simulink model "PubIfDecisionTOS_MDL"  (R2020b)
settings: configuration reference "DspaceConfig" (kept outside this file)
PostLoadFcn:
  | if any(exist('dsrtsu_mdlpostloadfcn', 'file') ~= 0), dsrtsu_mdlpostloadfcn('Execute', bdroot); end
InitFcn:
  | , if any(exist('dsmpb_private', 'file') ~= 0), dsmpb_private('dsmpb_mdlclblib', 'Init', bdroot); end,
undefined symbols (not defined in the file or in its folder): C_TOS_ACCEgoRAxletoFbumplength_m, C_TOS_ACCTargetFront_Flag, C_TOS_AEBJAPedObjDxThre_Val, C_TOS_AEBJAPedObjDyThre_Val, C_TOS_AEBJATargetSize_Val, C_TOS_AEBJAVehObjDxThre_Val, C_TOS_AEBJAVehObjDyThre_Val, C_TOS_AEBJuncPedTargetSize_Val, C_TOS_AEBLatObjDxThre_Val, C_TOS_AEBLatPedDyThre_Val, C_TOS_AEBLatTargetSize_Val, C_TOS_AEBLongTargetInEgoFront_Flag, C_TOS_axAbsGround_Parameter, C_TOS_CameraConfirmedFlag, C_TOS_CNsubjWidth, C_TOS_CurrentLaneCoreMinWidth_Val, C_TOS_CutInProb_Val_Zero, C_TOS_CutOutProb_Val_Zero, C_TOS_D2R_Val, C_TOS_DefaultValueObjectToCenterLine_dy, C_TOS_EgoCarWidth_Val, C_TOS_EgoDxRefPoint_m, C_TOS_EgoRAxletoFbumplength_m, C_TOS_HalfWidthVehicle_Con, C_TOS_HWA_CurrentLaneFlag, C_TOS_HWA_LeftLaneFlag, C_TOS_HWA_MovingDir_Vaild, C_TOS_HWA_MovState_Vaild, C_TOS_HWA_RightLaneFlag, C_TOS_LaneLineCourseErrorFront, C_TOS_LaneLineCourseErrorRear, C_TOS_MotorbikeDefaultWidth_m, C_TOS_NumberOfEffectiveTargets, C_TOS_Obj_Age_Val, C_TOS_Objdx_Constraint_Val, C_TOS_ObjectDefaultWidth_m, C_TOS_ObjInCurrentLane_Val, C_TOS_ObjInCurrentLaneValid, C_TOS_ObjInLeftLaneValid, C_TOS_ObjInRightLaneValid, C_TOS_ObjNotInCurrentLane_Val, C_TOS_ObjNotREElementType, C_TOS_ObjPredictDis_dy_ConstantVal_Zeros, C_TOS_ObjToCenterLine_ConstantVal_Zeros, C_TOS_OFMObjIDInvilad_Val, C_TOS_PIL_LatDisCons_Val_zero, C_TOS_PIL_ObjectCutInFlag_b, C_TOS_PIL_ObjectCutOutFlag_b, C_TOS_PIL_ObjLaneProb_al_Val, C_TOS_PP_ObjFusType_FC_Confirm_b, C_TOS_PP_ObjFusType_FC_FR_Confirm_b, C_TOS_PP_ObjFusType_FR_Confirm_b, C_TOS_RE_80BoolDefault_Val, C_TOS_RE_80Single181Default_Val, C_TOS_RE_80Single255Default_Val, C_TOS_RE_80Uint8Default_Val, C_TOS_RE_D2R, C_TOS_RE_D_180_Val, C_TOS_RE_InvalidObjectID_Val, C_TOS_RE_InvalidTargetChainDir_Val ... (+142)
libraries: simulink x1650, TOS_LIB x361, canfdmsglib x14
(part 3 of 69)

== system PubIfDecisionTOS_MDL/TOS_20201112/TOS_2012080320/Subsystem2 ==
  TOS_ACCP0 : Inport
  TOS_ACCP1 : Inport  Port=2
  TOS_ACCP2 : Inport  Port=3
  TOS_ACCP3 : Inport  Port=4
  TOS_ACC4 : Inport  Port=5
  TOS_ACCP5 : Inport  Port=6
  Bus Selector : BusSelector  OutputSignals=ACCTgtObjAy,ACCTgtObjCntAlive,ACCTgtObjExist,ACCTgtObjObstcl,ACCTgtObjVy,IDP0,ObjDYP0,ObjMovingStateP0,ObjTypeP0,Object_Orientation,P0CutInflg,P0HeadingAngle,axAbsGroundP0,dxP0,fu_typeP0,rangeP0,targetExistP0,vxRelP0
  Bus Selector1 : BusSelector  OutputSignals=IDP1,ObjDYP1,ObjMovingStateP1,ObjTypeP1,P1HeadingAngle,axAbsGroundP1,dxP1,fu_typeP1,rangeP1,targetExistP1,vxRelP1
  Bus Selector2 : BusSelector  OutputSignals=IDP2,ObjDYP2,ObjMovingStateP2,ObjTypeP2,P2CutinProb,P2HeadingAngle,axAbsGroundP2,dxP2,fu_typeP2,rangeP2,targetExistP2,vxRelP2
  Bus Selector3 : BusSelector  OutputSignals=IDP3,ObjDYP3,ObjMovingStateP3,ObjTypeP3,P3CutinProb,P3HeadingAngle,axAbsGroundP3,dxP3,fu_typeP3,rangeP3,targetExistP3,vxRelP3
  Bus Selector4 : BusSelector  OutputSignals=ObjTypeP4,dxP4,dyP4,targetExistP4
  Bus Selector5 : BusSelector  OutputSignals=ObjTypeP5,dxP5,dyP5,targetExistP5
  CAN FD Pack : canfdmsglib/CAN FD Pack  CANdbFile=F:\InternalData03_ACC_AEBLog_ELK_LC_LCKie_20200927.dbc  MsgList=(none)  MsgName=TOS_ACC_P0  ProtocolMode=CAN FD  MsgIDType=Standard (11-bit identifier)  MsgIdentifier=512  MsgLength=64  Remote=off  BRSSwitch=off  ApplyMinMax=off  SignalInfo={'{'P0_ACCTgtObjAy','12','12','BE','signed','Standard','0','0.01','0','-20.48','20.47';'P0_ACCTgtObjCntAlive','16','8','BE','unsigned','Standard','0','1','0','0','255';'P0_ACCTgtObjExist','24','8','BE','unsigned','Standard','0','0.01','0','0','2.55';'P0_ACCTgtObjObstcl','46','10','BE','unsigned','Standard','0','0.001','0','0','1.023';'P0_ACCTgtObjVy','58','14','BE','signed','Standard','0','0.01','0','-81.92','81.91';'P0_IDP0','96','8','BE','unsigned','Standard','0','1','0','0','255';'P0_ObjDYP0','114','14','BE','signed','Standard','0','0.005','0','-40.96','40.955';'P0_ObjMovingStateP0','122','6','BE','unsigned','Standard','0','1','0','0','63';'P0_ObjTypeP0','72','4','BE','unsigned','Standard','0','1','0','0','15';'P0_Object_Orientation','8','4','BE','unsigned','Standard','0','1','0','0','15';'P0_P0CutInflg','57','1','BE','unsigned','Standard','0','1','0','0','1';'P0_P0HeadingAngle','128','8','BE','unsigned','Standard','0','0.0041','0','0','1.0455';'P0_axAbsGroundP0','76','12','BE','signed','Standard','0','0.01','0','-20.48','20.47';'P0_dxP0','89','15','BE','unsigned','Standard','0','0.0063','0','0','206.4321';'P0_fu_typeP0','40','6','BE','unsigned','Standard','0','1','0','0','63';'P0_rangeP0','145','15','BE','unsigned','Standard','0','0.01','0','0','327.67';'P0_targetExistP0','56','1','BE','unsigned','Standard','0','1','0','0','1'}
      settings: SourceProductBaseCode=VN  DataFormat=CANdb specified signals
  CAN FD Pack1 : canfdmsglib/CAN FD Pack  CANdbFile=F:\InternalData03_ACC_AEBLog_ELK_LC_LCKie_20200927.dbc  MsgList=(none)  MsgName=TOS_ACC_P1_P2_P3_P4_P5  ProtocolMode=CAN FD  MsgIDType=Standard (11-bit identifier)  MsgIdentifier=513  MsgLength=64  Remote=off  BRSSwitch=off  ApplyMinMax=off  SignalInfo={'{'P1_IDP1','16','8','BE','unsigned','Standard','0','1','0','0','255';'P1_ObjDYP1','58','14','BE','signed','Standard','0','0.005','0','-40.96','40.955';'P1_ObjMovingStateP1','66','6','BE','unsigned','Standard','0','1','0','0','63';'P1_ObjTypeP1','32','4','BE','unsigned','Standard','0','1','0','0','15';'P1_P1HeadingAngle','72','8','BE','unsigned','Standard','0','0.0041','0','0','1.0455';'P1_axAbsGroundP1','36','12','BE','signed','Standard','0','0.01','0','-20.48','20.47';'P1_dxP1','9','15','BE','unsigned','Standard','0','0.0063','0','0','206.4321';'P1_fu_typeP1','42','6','BE','unsigned','Standard','0','1','0','0','63';'P1_rangeP1','89','15','BE','unsigned','Standard','0','0.0063','0','0','206.4321';'P1_targetExistP1','8','1','BE','unsigned','Standard','0','1','0','0','1';'P1_vxRelP1','104','16','BE','signed','Standard','0','0.00616','0','-201.8509','201.8447';'P2_IDP2','152','8','BE','unsigned','Standard','0','1','0','0','255';'P2_ObjDYP2','170','14','BE','signed','Standard','0','0.005','0','-40.96','40.955';'P2_ObjMovingStateP2','178','6','BE','unsigned','Standard','0','1','0','0','63';'P2_ObjTypeP2','120','4','BE','unsigned','Standard','0','1','0','0','15';'P2_P2CutinProb','184','8','BE','unsigned','Standard','0','0.005','0','0','1.275';'P2_P2HeadingAngle','192','8','BE','unsigned','Standard','0','0.0041','0','0','1.0455';'P2_axAbsGroundP2','124','12','BE','signed','Standard','0','0.01','0','-20.48','20.47';'P2_dxP2','137','15','BE','unsigned','Standard','0','0.0063','0','0','206.4321';'P2_fu_typeP2','146','6','BE','unsigned','Standard','0','1','0','0','63';'P2_rangeP2','209','15','BE','unsigned','Standard','0','0.0063','0','0','206.4321';'P2_targetExistP2','41','1','BE','unsigned','Standard','0','1','0','0','1';'P2_vxRelP2','232','16','BE','signed','Standard','0','0.00616','0','-201.8509','201.8447';'P3_IDP3','272','8','BE','unsigned','Standard','0','1','0','0','255';'P3_ObjDYP3','290','14','BE','signed','Standard','0','0.005','0','-40.96','40.955';'P3_ObjMovingStateP3','298','6','BE','unsigned','Standard','0','1','0','0','63';'P3_ObjTypeP3','248','4','BE','unsigned','Standard','0','1','0','0','15';'P3_P3CutinProb','304','8','BE','unsigned','Standard','0','0.005','0','0','1.275';'P3_P3HeadingAngle','312','8','BE','unsigned','Standard','0','0.0041','0','0','1.0455';'P3_axAbsGroundP3','252','12','BE','signed','Standard','0','0.01','0','-20.48','20.47';'P3_dxP3','265','15','BE','unsigned','Standard','0','0.0063','0','0','206.4321';'P3_fu_typeP3','218','6','BE','unsigned','Standard','0','1','0','0','63';'P3_rangeP3','329','15','BE','unsigned','Standard','0','0.0063','0','0','206.4321';'P3_targetExistP3','40','1','BE','unsigned','Standard','0','1','0','0','1';'P3_vxRelP3','344','16','BE','signed','Standard','0','0.00616','0','-201.8509','201.8447';'P4_ObjTypeP4','376','4','BE','unsigned','Standard','0','1','0','0','15';'P4_dxP4','361','15','BE','unsigned','Standard','0','0.0063','0','0','206.4321';'P4_dyP4','380','12','BE','signed','Standard','0','0.01','0','-20.48','20.47';'P4_targetExistP4','57','1','BE','unsigned','Standard','0','1','0','0','1';'P5_ObjTypeP5','408','4','BE','unsigned','Standard','0','1','0','0','15';'P5_dxP5','393','15','BE','unsigned','Standard','0','0.0063','0','0','206.4321';'P5_dyP5','412','12','BE','signed','Standard','0','0.01','0','-20.48','20.47'}
      settings: SourceProductBaseCode=VN  DataFormat=CANdb specified signals
  TOS_ACCP0_Msg : Outport
  TOS_ACCP1_P2_P3_P4_P5_Msg : Outport  Port=2
  wires:
  TOS_ACCP2/1 -> Bus Selector2/1
  TOS_ACCP1/1 -> Bus Selector1/1
  TOS_ACCP0/1 -> Bus Selector/1
  CAN FD Pack/1 -> TOS_ACCP0_Msg/1
  TOS_ACCP3/1 -> Bus Selector3/1
  TOS_ACC4/1 -> Bus Selector4/1
  TOS_ACCP5/1 -> Bus Selector5/1
  Bus Selector/1 -> CAN FD Pack/1  "<ACCTgtObjAy>"
  Bus Selector/2 -> CAN FD Pack/2  "<ACCTgtObjCntAlive>"
  Bus Selector/3 -> CAN FD Pack/3  "<ACCTgtObjExist>"
  Bus Selector/4 -> CAN FD Pack/4  "<ACCTgtObjObstcl>"
  Bus Selector/5 -> CAN FD Pack/5  "<ACCTgtObjVy>"
  Bus Selector/6 -> CAN FD Pack/6  "<IDP0>"
  Bus Selector/7 -> CAN FD Pack/7  "<ObjDYP0>"
  Bus Selector/8 -> CAN FD Pack/8  "<ObjMovingStateP0>"
  Bus Selector/9 -> CAN FD Pack/9  "<ObjTypeP0>"
  Bus Selector/10 -> CAN FD Pack/10  "<Object_Orientation>"
  Bus Selector/11 -> CAN FD Pack/11  "<P0CutInflg>"
  Bus Selector/12 -> CAN FD Pack/12  "<P0HeadingAngle>"
  Bus Selector/13 -> CAN FD Pack/13  "<axAbsGroundP0>"
  Bus Selector/14 -> CAN FD Pack/14  "<dxP0>"
  Bus Selector/15 -> CAN FD Pack/15  "<fu_typeP0>"
  Bus Selector/16 -> CAN FD Pack/16  "<rangeP0>"
  Bus Selector/17 -> CAN FD Pack/17  "<targetExistP0>"
  Bus Selector/18 -> CAN FD Pack/18  "<vxRelP0>"
  Bus Selector1/4 -> CAN FD Pack1/4  "<ObjTypeP1>"
  Bus Selector1/5 -> CAN FD Pack1/5  "<P1HeadingAngle>"
  Bus Selector1/3 -> CAN FD Pack1/3  "<ObjMovingStateP1>"
  Bus Selector1/6 -> CAN FD Pack1/6  "<axAbsGroundP1>"
  Bus Selector1/2 -> CAN FD Pack1/2  "<ObjDYP1>"
  Bus Selector1/7 -> CAN FD Pack1/7  "<dxP1>"
  Bus Selector1/1 -> CAN FD Pack1/1  "<IDP1>"
  Bus Selector1/8 -> CAN FD Pack1/8  "<fu_typeP1>"
  Bus Selector1/9 -> CAN FD Pack1/9  "<rangeP1>"
  Bus Selector1/10 -> CAN FD Pack1/10  "<targetExistP1>"
  Bus Selector1/11 -> CAN FD Pack1/11  "<vxRelP1>"
  Bus Selector2/4 -> CAN FD Pack1/15  "<ObjTypeP2>"
  Bus Selector2/5 -> CAN FD Pack1/16  "<P2CutinProb>"
  Bus Selector2/3 -> CAN FD Pack1/14  "<ObjMovingStateP2>"
  Bus Selector2/6 -> CAN FD Pack1/17  "<P2HeadingAngle>"
  Bus Selector2/2 -> CAN FD Pack1/13  "<ObjDYP2>"
  Bus Selector2/7 -> CAN FD Pack1/18  "<axAbsGroundP2>"
  Bus Selector2/1 -> CAN FD Pack1/12  "<IDP2>"
  Bus Selector2/8 -> CAN FD Pack1/19  "<dxP2>"
  Bus Selector2/9 -> CAN FD Pack1/20  "<fu_typeP2>"
  Bus Selector2/10 -> CAN FD Pack1/21  "<rangeP2>"
  Bus Selector2/11 -> CAN FD Pack1/22  "<targetExistP2>"
  Bus Selector2/12 -> CAN FD Pack1/23  "<vxRelP2>"
  Bus Selector3/1 -> CAN FD Pack1/24  "<IDP3>"
  Bus Selector3/2 -> CAN FD Pack1/25  "<ObjDYP3>"
  Bus Selector3/3 -> CAN FD Pack1/26  "<ObjMovingStateP3>"
  Bus Selector3/4 -> CAN FD Pack1/27  "<ObjTypeP3>"
  Bus Selector3/5 -> CAN FD Pack1/28  "<P3CutinProb>"
  Bus Selector3/6 -> CAN FD Pack1/29  "<P3HeadingAngle>"
  Bus Selector3/7 -> CAN FD Pack1/30  "<axAbsGroundP3>"
  Bus Selector3/8 -> CAN FD Pack1/31  "<dxP3>"
  Bus Selector3/9 -> CAN FD Pack1/32  "<fu_typeP3>"
  Bus Selector3/10 -> CAN FD Pack1/33  "<rangeP3>"
  Bus Selector3/11 -> CAN FD Pack1/34  "<targetExistP3>"
  Bus Selector3/12 -> CAN FD Pack1/35  "<vxRelP3>"
  Bus Selector4/3 -> CAN FD Pack1/38  "<dyP4>"
  Bus Selector4/2 -> CAN FD Pack1/37  "<dxP4>"
  Bus Selector4/4 -> CAN FD Pack1/39  "<targetExistP4>"
  Bus Selector4/1 -> CAN FD Pack1/36  "<ObjTypeP4>"
  Bus Selector5/1 -> CAN FD Pack1/40  "<ObjTypeP5>"
  Bus Selector5/2 -> CAN FD Pack1/41  "<dxP5>"
  Bus Selector5/3 -> CAN FD Pack1/42  "<dyP5>"
  Bus Selector5/4 -> CAN FD Pack1/43  "<targetExistP5>"
  CAN FD Pack1/1 -> TOS_ACCP1_P2_P3_P4_P5_Msg/1
